simulink model "PIUIOModel"  (R2016a)
settings: Solver=VariableStepAuto  StartTime=0.0  StopTime=tEnd  RelTol=1e-3
values from neighbouring files (symbols this model uses):
  A = [-1 1 1;1 -2 0;0 1 -3]    [ExampleActuator.m]    (also in ExamplePIUIO.m = [-2 0 1;0 -1 1;1 2 -3]; NewExampleActuator.m; Simulation.m; SinousidPIUIO.m)
  B = [1;1;0]    [ExampleActuator.m]    (also in ExamplePIUIO.m = [1;0;1]; NewExampleActuator.m; Simulation.m; SinousidPIUIO.m)
  C = [1 0 0;0 1 0]    [ExampleActuator.m]    (also in ExamplePIUIO.m = [1 2 3;0 1 2]; NewExampleActuator.m = [1 0 1;0 1 0]; Simulation.m = [1 0 1;0 1 0]; SinousidPIUIO.m = [1 0 1;0 1 0])
  d = dTS.Values.Data    [ExampleActuator.m]    (also in ExamplePIUIO.m; NewExampleActuator.m = 2; Simulation.m; SinousidPIUIO.m = 1)
  Ea = [1;0;1]    [ExamplePIUIO.m]    (also in Simulation.m = [1;1;0]; SinousidPIUIO.m = [1;0;0])
  Ed = [1;0;0]    [ExampleActuator.m]    (also in ExamplePIUIO.m = [1;1;0]; NewExampleActuator.m; Simulation.m; SinousidPIUIO.m = [1;0;1])
  fa = faTS.Values.Data    [ExamplePIUIO.m]    (also in Simulation.m = 3; SinousidPIUIO.m)
  fahat0 = [5]    [ExamplePIUIO.m]    (also in SinousidPIUIO.m = [1])
  G1 = P\Y    [ExampleActuator.m]    (also in ExamplePIUIO.m = Lhat(1:n,:); NewExampleActuator.m = (place(A1',C',observerPoles))'; PUIOfinder.m; SinousidPIUIO.m = Lhat(1:n,:))
  J = T*Ea    [ExamplePIUIO.m]    (also in SinousidPIUIO.m)
  L = Lhat(n+1:end,:)    [ExamplePIUIO.m]    (also in SinousidPIUIO.m)
  N = Ed* pinv(C*Ed)    [ExampleActuator.m]    (also in ExamplePIUIO.m; NewExampleActuator.m; PUIOfinder.m = E* pinv(C*E); SinousidPIUIO.m)
  R = 0    [ExamplePIUIO.m]    (also in SinousidPIUIO.m = -3)
  x0 = [1;2;3]    [ExampleActuator.m]    (also in ExamplePIUIO.m; NewExampleActuator.m; Simulation.m; SinousidPIUIO.m)
  xhat0 = [2;1;1]    [ExamplePIUIO.m]    (also in Simulation.m = [.1;.2;.3;.4;.5]; SinousidPIUIO.m)
settings Model: Creator=amirreza513  LastModifiedBy=amirreza513

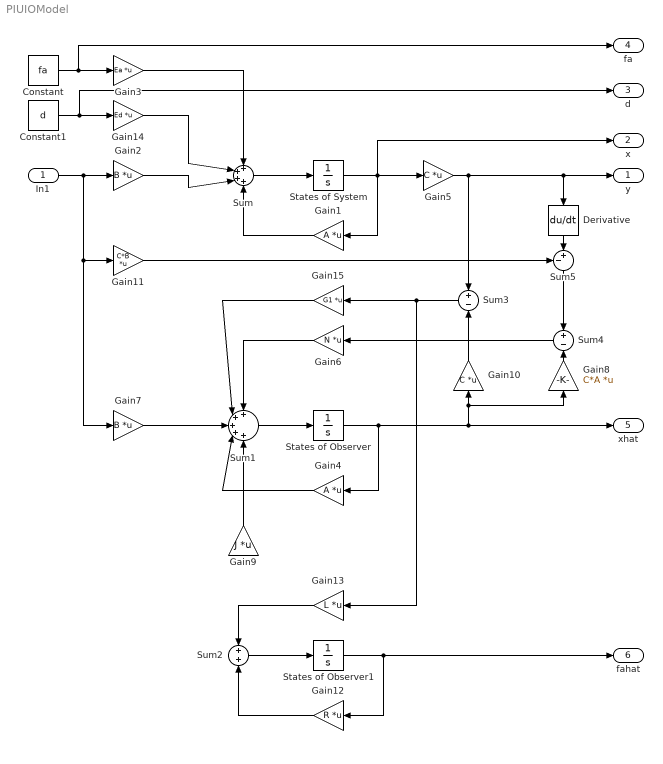
== system PIUIOModel ==
  In1 : Inport
  Constant : Constant  Value=fa
  Constant1 : Constant  Value=d
  Derivative : Derivative  CoefficientInTFapproximation=0
  Gain1 : Gain  Gain=A  Multiplication=Matrix(K*u) (u vector)
  Gain10 : Gain  Gain=C  Multiplication=Matrix(K*u) (u vector)
  Gain11 : Gain  Gain=C*B  Multiplication=Matrix(K*u) (u vector)
  Gain12 : Gain  Gain=R  Multiplication=Matrix(K*u) (u vector)
  Gain13 : Gain  Gain=L  Multiplication=Matrix(K*u) (u vector)
  Gain14 : Gain  Gain=Ed  Multiplication=Matrix(K*u) (u vector)
  Gain15 : Gain  Gain=G1  Multiplication=Matrix(K*u) (u vector)
  Gain2 : Gain  Gain=B  Multiplication=Matrix(K*u) (u vector)
  Gain3 : Gain  Gain=Ea  Multiplication=Matrix(K*u) (u vector)
  Gain4 : Gain  Gain=A  Multiplication=Matrix(K*u) (u vector)
  Gain5 : Gain  Gain=C  Multiplication=Matrix(K*u) (u vector)
  Gain6 : Gain  Gain=N  Multiplication=Matrix(K*u) (u vector)
  Gain7 : Gain  Gain=B  Multiplication=Matrix(K*u) (u vector)
  Gain8 : Gain  Gain=C*A  Multiplication=Matrix(K*u) (u vector)
  Gain9 : Gain  Gain=J  Multiplication=Matrix(K*u) (u vector)
  States of Observer : Integrator  InitialCondition=xhat0
  States of Observer1 : Integrator  InitialCondition=fahat0
  States of System : Integrator  InitialCondition=x0
  Sum : Sum  Inputs=++++
  Sum1 : Sum  Inputs=+++++
  Sum2 : Sum
  Sum3 : Sum  Inputs=+-
  Sum4 : Sum  Inputs=+-
  Sum5 : Sum  Inputs=-+|
  y : Outport
  x : Outport  Port=2
  d : Outport  Port=3
  fa : Outport  Port=4
  xhat : Outport  Port=5
  fahat : Outport  Port=6
  wires:
  States of System/1 -> x/1, Gain5/1, Gain1/1
  In1/1 -> Gain7/1, Gain11/1, Gain2/1
  Constant/1 -> fa/1, Gain3/1
  Sum/1 -> States of System/1
  Gain5/1 -> Sum3/1, Derivative/1, y/1
  Gain3/1 -> Sum/1
  Sum1/1 -> States of Observer/1
  States of Observer/1 -> xhat/1, Gain8/1, Gain10/1, Gain4/1
  Constant1/1 -> Gain14/1, d/1
  Gain14/1 -> Sum/2
  Gain2/1 -> Sum/3
  Gain1/1 -> Sum/4
  Gain7/1 -> Sum1/3
  Gain4/1 -> Sum1/4
  Sum3/1 -> Gain13/1, Gain15/1
  Gain10/1 -> Sum3/2
  Gain15/1 -> Sum1/2
  Gain6/1 -> Sum1/1
  Sum4/1 -> Gain6/1
  Gain8/1 -> Sum4/2
  Derivative/1 -> Sum5/2
  Gain11/1 -> Sum5/1
  Sum5/1 -> Sum4/1
  Gain9/1 -> Sum1/5
  States of Observer1/1 -> Gain12/1, fahat/1
  Sum2/1 -> States of Observer1/1
  Gain12/1 -> Sum2/2
  Gain13/1 -> Sum2/1
